simulink model "week5_inclass_pp_v_1"  (R2020b)
settings: Solver=FixedStepAuto  StartTime=0.0  StopTime=Ts  FixedStep=0.1  RelTol=1e-3
InitFcn:
  | pure_pusuit_inclass_init
StopFcn:
  | simulation_plots_week5
values from neighbouring files (symbols this model uses):
  L = 3    [lateral_vehicle_animation.m]    (also in trajectory_plot_lanechange.m = wheel_base)
undefined symbols (not defined in the file or in its folder): ld, vRef, xRef, yRef
libraries: autolibshared x1, robotalgslib x1
settings Model: Creator=anime  LastModifiedBy=anime

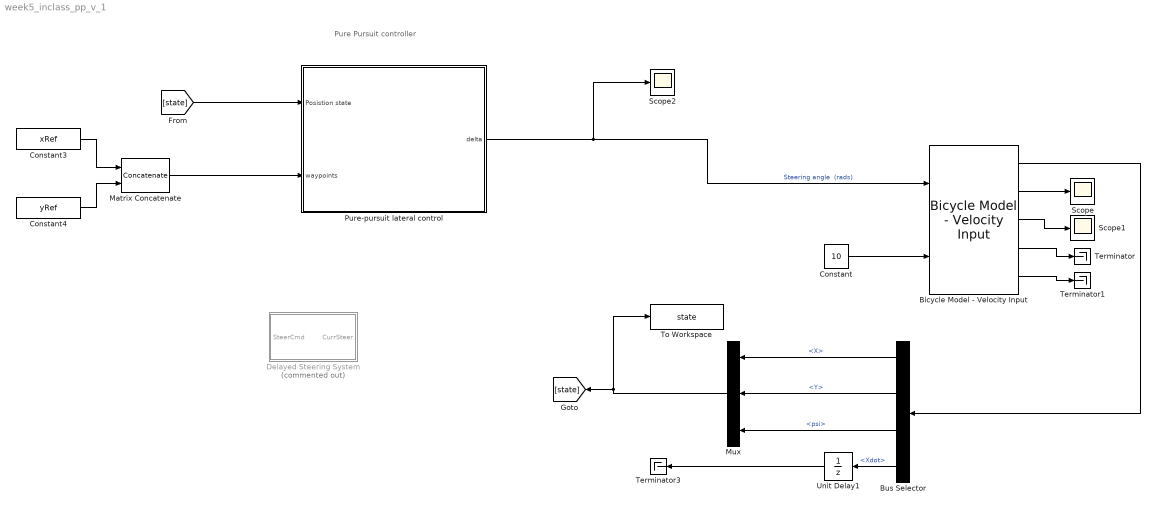
== system week5_inclass_pp_v_1 ==
  note: Pure Pursuit controller
  Bicycle Model - Velocity Input : autolibshared/Bicycle Model - Velocity Input  trackMode=Single (bicycle)  inputMode=External longitudinal forces  frontSteerMode=on  rearSteerMode=off  windMode=off  muMode=off  extFMode=off  extMMode=off  aMode=3  NF=2  NR=2  m=1575  a=1.2  b=1.6  h=0.35  X_o=X_o  xdot_o=0  CalphaMode=off  sigmaMode=on  w=[1.4,1.4]  Cy_f=19e3  Cy_r=20e3  sigma_f=.1  sigma_r=.1  alpha_f_brk=[-.1 .1]  Cy_f_data=[-9e3 9e3]  alpha_r_brk=[-.1 .1]  Cy_r_data=[-9e3 9e3]  Y_o=Y_o  ydot_o=0  Izz=4000  psi_o=psi_o  r_o=0  Af=2  Cd=.3  Cl=.1  Cpm=.1  beta_w=[0:0.01:0.3]  Cs=[0:0.03:0.9]  Cym=[0:0.01:0.3]  Pabs=101325  Tair=273  g=9.81  mu=1  xdot_tol=.01  Fznom=5000  Fxtire_sat=1e6  Fytire_sat=1e6  longOff=0  latOff=0  vertOff=0
      settings: SourceProductBaseCode=PW,MT,UV,VE,VP
  Bus Selector : BusSelector  OutputSignals=InertFrm.Cg.Disp.X,InertFrm.Cg.Disp.Y,InertFrm.Cg.Ang.psi,InertFrm.Cg.Vel.Xdot
  Constant : Constant  Value=10
  Constant3 : Constant  Value=xRef  SampleTime=0.1
  Constant4 : Constant  Value=yRef  SampleTime=0.1
  Delayed Steering System : Subsystem  Commented=on
  Matrix Concatenate : Concatenate  Mode=Multidimensional array  ConcatenateDimension=2
  Mux : Mux  Inputs=3
  Pure-pursuit lateral control : Subsystem
  Scope : Scope
  Scope1 : Scope
  Scope2 : Scope
  Terminator : Terminator
  Terminator1 : Terminator
  Terminator3 : Terminator
  To Workspace : ToWorkspace  VariableName=state  SampleTime=-1
  Unit Delay1 : UnitDelay  InitialCondition=vRef  SampleTime=-1  HasFrameUpgradeWarning=on
  wires:
  Constant4/1 -> Matrix Concatenate/2
  Constant3/1 -> Matrix Concatenate/1
  Constant/1 -> Bicycle Model - Velocity Input/2
  Bicycle Model - Velocity Input/2 -> Scope/1
  Bicycle Model - Velocity Input/3 -> Scope1/1
  Bicycle Model - Velocity Input/4 -> Terminator/1
  Bicycle Model - Velocity Input/5 -> Terminator1/1
  [state] -> Pure-pursuit lateral control/1(Posistion state)
  Matrix Concatenate/1 -> Pure-pursuit lateral control/2(waypoints)
  Pure-pursuit lateral control/1(delta) -> Scope2/1, Bicycle Model - Velocity Input/1  "Steering angle  (rads)"
  Unit Delay1/1 -> Terminator3/1
  Bus Selector/2 -> Mux/2  "<Y>"
  Bus Selector/4 -> Unit Delay1/1  "<Xdot>"
  Bicycle Model - Velocity Input/1 -> Bus Selector/1
  Mux/1 -> To Workspace/1, [state]
  Bus Selector/1 -> Mux/1  "<X>"
  Bus Selector/3 -> Mux/3  "<psi>"

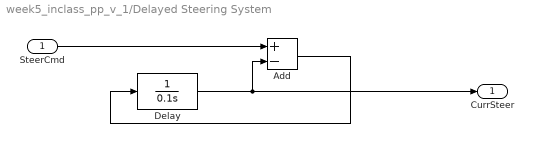
== system week5_inclass_pp_v_1/Delayed Steering System ==
  SteerCmd : Inport
  Add : Sum  Inputs=+-
  Delay : TransferFcn  Denominator=[0.1 0]
  CurrSteer : Outport  VectorParamsAs1DForOutWhenUnconnected=off
  wires:
  Add/1 -> Delay/1
  SteerCmd/1 -> Add/1
  Delay/1 -> CurrSteer/1, Add/2

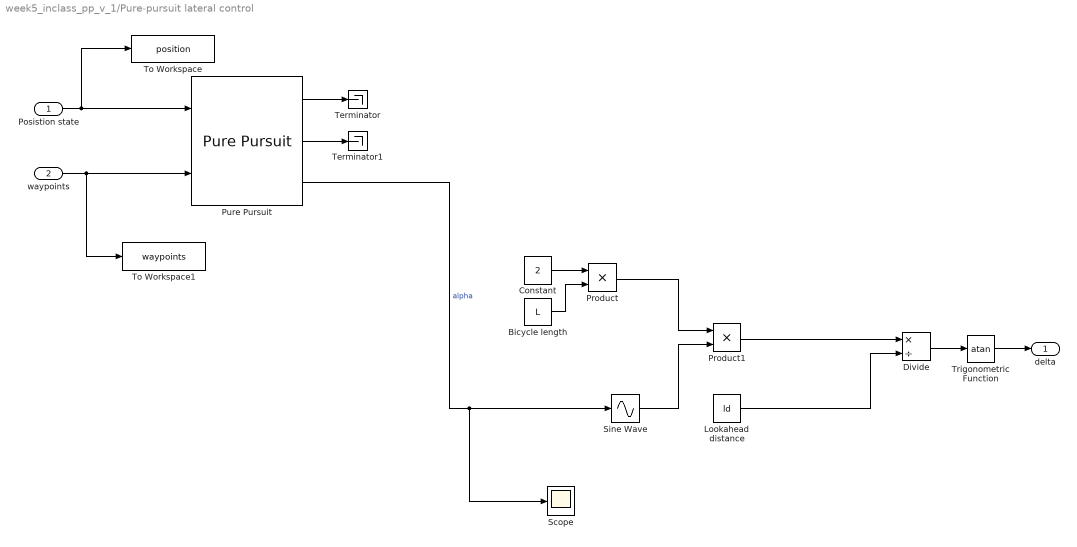
== system week5_inclass_pp_v_1/Pure-pursuit lateral control ==
  Posistion state : Inport
  waypoints : Inport  Port=2
  Bicycle length : Constant  Value=L
  Constant : Constant  Value=2
  Divide : Product  Inputs=*/
  Lookahead distance : Constant  Value=ld
  Product : Product
  Product1 : Product
  Pure Pursuit : robotalgslib/Pure Pursuit  DesiredLinearVelocity=vRef  MaxAngularVelocity=inf  LookaheadDistance=ld  TargetDirPort=on  SimulateUsing=Code generation
  Scope : Scope
  Sine Wave : Sin  TimeSource=Use external signal  SampleTime=0
  Terminator : Terminator
  Terminator1 : Terminator
  To Workspace : ToWorkspace  VariableName=position  SampleTime=-1
  To Workspace1 : ToWorkspace  VariableName=waypoints  SampleTime=-1
  Trigonometric Function : Trigonometry  Operator=atan
  delta : Outport
  wires:
  Posistion state/1 -> To Workspace/1, Pure Pursuit/1
  waypoints/1 -> To Workspace1/1, Pure Pursuit/2
  Pure Pursuit/1 -> Terminator/1
  Pure Pursuit/2 -> Terminator1/1
  Trigonometric Function/1 -> delta/1
  Constant/1 -> Product/1
  Divide/1 -> Trigonometric Function/1
  Lookahead distance/1 -> Divide/2
  Sine Wave/1 -> Product1/2
  Product1/1 -> Divide/1
  Pure Pursuit/3 -> Scope/1, Sine Wave/1  "alpha"
  Bicycle length/1 -> Product/2
  Product/1 -> Product1/1
